simulink model "Tabela_3_4"  (R2016a)
settings: Solver=VariableStepAuto  StartTime=0.0  StopTime=5/60  RelTol=1e-3
libraries: powerlib x14, dspstat3 x9
settings Model: Creator=55329  LastModifiedBy=55329

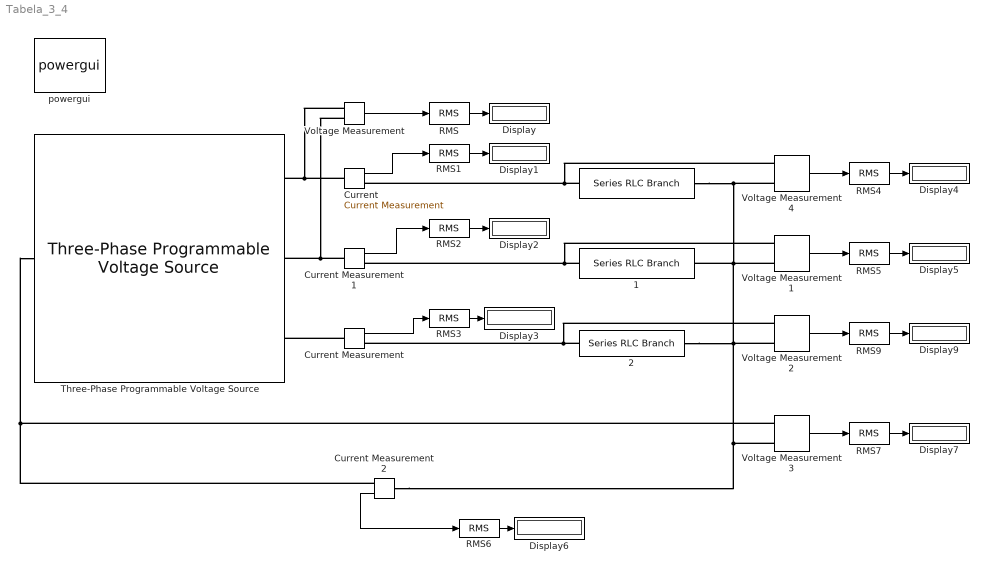
== system Tabela_3_4 ==
  " " : powerlib/Elements/Series RLC Branch  LConnTagsString=__new0  RConnTagsString=__new0  BranchType=R  Resistance=100  Inductance=1e-3  SetiL0=off  InitialCurrent=0  Capacitance=25e-6  Setx0=off  InitialVoltage=0  Measurements=None
  " 1" : powerlib/Elements/Series RLC Branch  LConnTagsString=__new0  RConnTagsString=__new0  BranchType=RC  Resistance=100  Inductance=1e-3  SetiL0=off  InitialCurrent=0  Capacitance=25e-6  Setx0=off  InitialVoltage=0  Measurements=None
  2 : powerlib/Elements/Series RLC Branch  LConnTagsString=__new0  RConnTagsString=__new0  BranchType=RC  Resistance=100  Inductance=1e-3  SetiL0=off  InitialCurrent=0  Capacitance=25e-6  Setx0=off  InitialVoltage=0  Measurements=None
  "Current " : powerlib/Measurements/Current Measurement  PhasorSimulation=off  OutputType=Complex  PSBequivalent=0
  Current Measurement : powerlib/Measurements/Current Measurement  PhasorSimulation=off  OutputType=Complex  PSBequivalent=0
  Current Measurement1 : powerlib/Measurements/Current Measurement  PhasorSimulation=off  OutputType=Complex  PSBequivalent=0
  Current Measurement2 : powerlib/Measurements/Current Measurement  PhasorSimulation=off  OutputType=Complex  PSBequivalent=0
  Display{,1..7,9} (9 alike) : Display
  RMS{,1..7,9} (9 alike) : dspstat3/RMS  run=on  reset_popup=None  InputProcessing=Columns as channels (frame based)  directionMode=Each column  dimension=1
  Three-Phase Programmable Voltage Source : powerlib/Electrical Sources/Three-Phase Programmable Voltage Source  PositiveSequence="[220  0 60]"  VariationEntity=None  VariationType=Table of time-amplitude pairs  VariationTypeAlt=Modulation  VariationStep=0.5  VariationRate=10  VariationMagnitude=0.3  VariationFrequency=2  VariationTiming=[1 2]  VariationPhaseA=off  Amplitudes=[1 0.8 1.2 1.0]  TimeValues=[0 0.1 0.15 0.2]  HarmonicGeneration=off  HarmonicA=[3 0.2 -25 0]  HarmonicB=[2 0.15 35 2]  Timing="[0.05  3]"  BusType=swing  Pref=0  Qref=0  Qmin=-inf  Qmax=inf
  Voltage Measurement{,1..4} (5 alike) : powerlib/Measurements/Voltage Measurement  PhasorSimulation=off  OutputType=Complex  PSBequivalent=0
  powergui : powerlib/powergui  Priority=1  SimulationMode=Discrete  SolverType=Tustin/Backward Euler (TBE)  SampleTime=50e-6  frequency=60  SPID=off  DisableSnubberDevices=off  DisableRonSwitches=off  DisableVfSwitches=off  SwTol=0  DisplayEquations=off  Interpol=off  ExternalGateDelay=off  methode=off  Ts=10  FunctionMessages=off  echomessages=off  HookPort=off  EnableUseOfTLC=off  x0status=blocks  frequencyindice=60  Pbase=100e6  ErrMax=1e-4  Iterations=50  UnitsV=kV  UnitsW=MW  buscounter=0  RestoreLinks=warning  ResistiveCurrentMeasurement=off  Frange=[0:2:500]  Ylog=off  Xlog=on  ShowGrid=off  save=off  variable=ZData  structure=0  ZoomFFT=off  StartTime=0.0  cycles=1  DisplayStyle=1  fundamental=60  FreqAxis=off  MaxFrequency=1000  frequencyindicesteady=1  RmsSteady=1  display=off
  wires:
  RMS1/1 -> Display1/1
  RMS/1 -> Display/1
  RMS2/1 -> Display2/1
  RMS3/1 -> Display3/1
  RMS4/1 -> Display4/1
  RMS5/1 -> Display5/1
  "Current "/1 -> RMS1/1
  Current Measurement1/1 -> RMS2/1
  Current Measurement/1 -> RMS3/1
  Voltage Measurement/1 -> RMS/1
  Voltage Measurement1/1 -> RMS5/1
  Voltage Measurement4/1 -> RMS4/1
  RMS9/1 -> Display9/1
  Voltage Measurement2/1 -> RMS9/1
  RMS7/1 -> Display7/1
  Voltage Measurement3/1 -> RMS7/1
  RMS6/1 -> Display6/1
  Current Measurement2/1 -> RMS6/1
  connections:
  Current Measurement/LConn1 -- Three-Phase Programmable Voltage Source/RConn3
  Current Measurement1/LConn1 -- Voltage Measurement/LConn2 -- Three-Phase Programmable Voltage Source/RConn2
  "Current "/LConn1 -- Voltage Measurement/LConn1 -- Three-Phase Programmable Voltage Source/RConn1
  " 1"/LConn1 -- Current Measurement1/RConn1 -- Voltage Measurement1/LConn1
  2/LConn1 -- Voltage Measurement2/LConn1 -- Current Measurement/RConn1
  " "/LConn1 -- Voltage Measurement4/LConn1 -- "Current "/RConn1
  2/RConn1 -- Current Measurement2/LConn1 -- Voltage Measurement3/LConn2 -- Voltage Measurement2/LConn2 -- Voltage Measurement1/LConn2 -- Voltage Measurement4/LConn2 -- " "/RConn1 -- " 1"/RConn1
  Voltage Measurement3/LConn1 -- Current Measurement2/RConn1 -- Three-Phase Programmable Voltage Source/LConn1
